simulink model "Step"  (R2023a)
settings: Solver=ode45  StartTime=0.0  StopTime=3.0  MaxStep=0.001  RelTol=1e-6  AbsTol=1e-6
values from neighbouring files (symbols this model uses):
  B = 30.2*0.137*60/(1000*7580*2*pi)    (= 5.21230338957e-06)    [Mechatronics.m]
  J = 142/(1000*100*100)    (= 1.42e-05)    [Mechatronics.m]
  Kp = 1    [Mechatronics.m]
  Kt = 30.2/1000    (= 0.0302)    [Mechatronics.m]
  Kw = 60/(317*2*pi)    (= 0.0301239639922)    [Mechatronics.m]
  L = 0.0823/1000    (= 8.23e-05)    [Mechatronics.m]
  R = 0.299    [Mechatronics.m]
settings Model: Creator=karteek  LastModifiedBy=karteek
settings DataIOCC: SaveOutput=off  SignalLogging=off  DSMLogging=off  SaveTime=off  ReturnWorkspaceOutputs=off

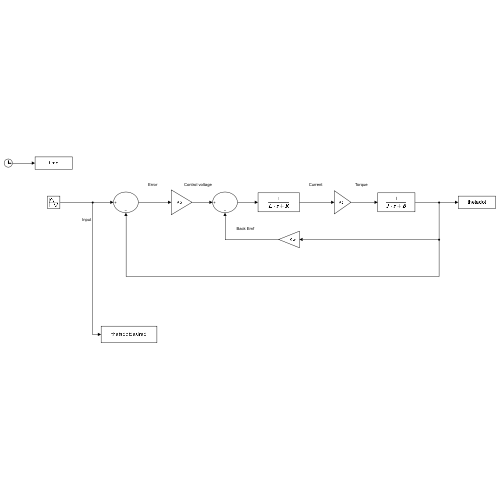
[thumbnail: Simulink's stored preview of the top-level diagram]
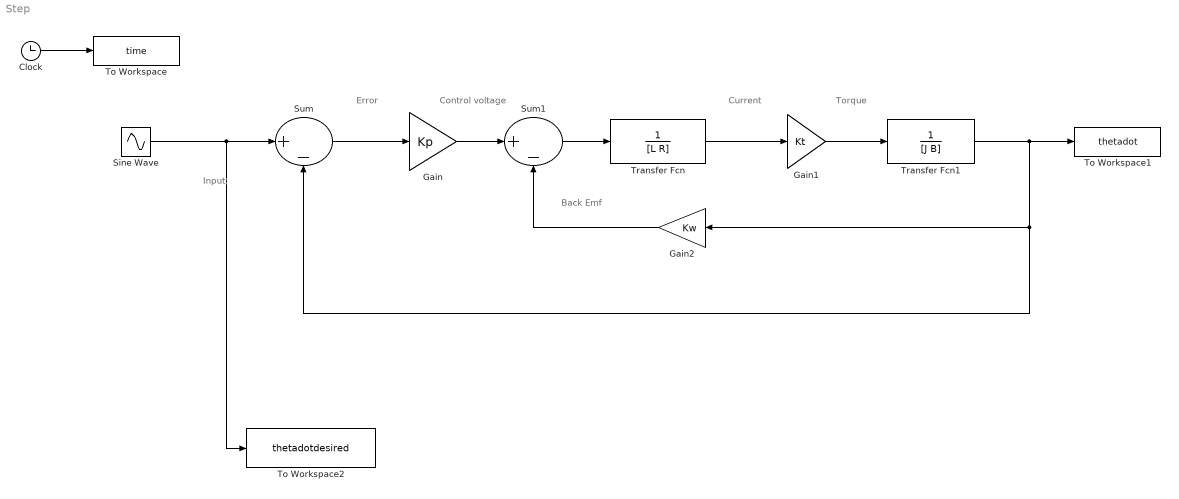
== system Step ==
  note: Torque
  note: Current
  note: Back Emf
  note: Control voltage
  note: Error
  note: Input
  Clock : Clock
  Gain : Gain  Gain=Kp
  Gain1 : Gain  Gain=Kt
  Gain2 : Gain  Gain=Kw
  Sine Wave : Sin  Amplitude=1000*2*pi/60  Bias=4000*2*pi/60  Frequency=6*pi  SampleTime=0
  Sum : Sum  Inputs=|+-
  Sum1 : Sum  Inputs=|+-
  To Workspace : ToWorkspace  VariableName=time  SampleTime=-1
  To Workspace1 : ToWorkspace  VariableName=thetadot  SampleTime=-1
  To Workspace2 : ToWorkspace  VariableName=thetadotdesired  SampleTime=-1
  Transfer Fcn : TransferFcn  Denominator=[L R]
  Transfer Fcn1 : TransferFcn  Denominator=[J B]
  wires:
  Sum/1 -> Gain/1
  Gain/1 -> Sum1/1
  Sum1/1 -> Transfer Fcn/1
  Transfer Fcn/1 -> Gain1/1
  Gain1/1 -> Transfer Fcn1/1
  Gain2/1 -> Sum1/2
  Transfer Fcn1/1 -> Gain2/1, Sum/2, To Workspace1/1
  Clock/1 -> To Workspace/1
  Sine Wave/1 -> Sum/1, To Workspace2/1
